simulink model "model_decouple_V0"  (R2020b)
settings: Solver=VariableStepAuto  StartTime=0.0  StopTime=10.0  RelTol=1e-3
values from neighbouring files (symbols this model uses):
  Px_e = xSeq    (= 0)    [Valeur_Equilibre.m]
  Py_e = ySeq    (= 0)    [Valeur_Equilibre.m]
  Vx_e = 0    [Valeur_Equilibre.m]
  Vy_e = 0    [Valeur_Equilibre.m]
  zD_e = Pzeq - XD*Ayeq + YD*Axeq    [Valeur_Equilibre.m]
  zE_e = Pzeq - XE*Ayeq + YE*Axeq    [Valeur_Equilibre.m]
  zF_e = Pzeq - XF*Ayeq + YF*Axeq    [Valeur_Equilibre.m]
undefined symbols (not defined in the file or in its folder): A_Ax, A_Ay, A_Az, A_Px, A_Py, B_Ax, B_Ay, B_Az, B_Px, B_Py, C_Ax, C_Ay, C_Az, C_Px, C_Py, D_Ax, D_Ay, D_Az, D_Px, D_Py, XA, XB, XC, XD, XE, XF, YB, YC, YD, YE, YF
settings Model: Creator=Alexi  LastModifiedBy=Alexi

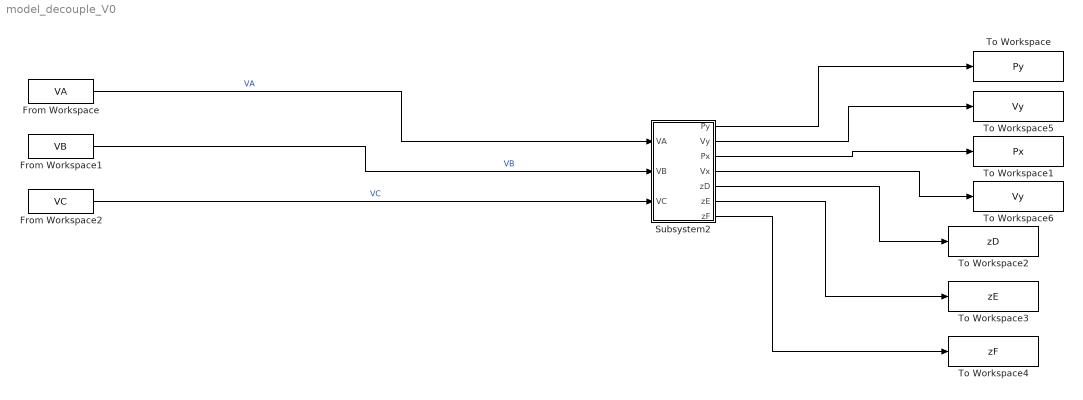
== system model_decouple_V0 ==
  From Workspace : FromWorkspace  VariableName=VA
  From Workspace1 : FromWorkspace  VariableName=VB
  From Workspace2 : FromWorkspace  VariableName=VC
  Subsystem2 : Subsystem
  To Workspace : ToWorkspace  VariableName=Py  SaveFormat=Timeseries  SampleTime=-1
  To Workspace1 : ToWorkspace  VariableName=Px  SaveFormat=Timeseries  SampleTime=-1
  To Workspace2 : ToWorkspace  VariableName=zD  SaveFormat=Timeseries  SampleTime=-1
  To Workspace3 : ToWorkspace  VariableName=zE  SaveFormat=Timeseries  SampleTime=-1
  To Workspace4 : ToWorkspace  VariableName=zF  SaveFormat=Timeseries  SampleTime=-1
  To Workspace5 : ToWorkspace  VariableName=Vy  SaveFormat=Timeseries  SampleTime=-1
  To Workspace6 : ToWorkspace  VariableName=Vy  SaveFormat=Timeseries  SampleTime=-1
  wires:
  From Workspace/1 -> Subsystem2/1(VA)  "VA"
  From Workspace1/1 -> Subsystem2/2(VB)  "VB"
  From Workspace2/1 -> Subsystem2/3(VC)  "VC"
  Subsystem2/1(Py) -> To Workspace/1
  Subsystem2/3(Px) -> To Workspace1/1
  Subsystem2/5(zD) -> To Workspace2/1
  Subsystem2/6(zE) -> To Workspace3/1
  Subsystem2/7(zF) -> To Workspace4/1
  Subsystem2/2(Vy) -> To Workspace5/1
  Subsystem2/4(Vx) -> To Workspace6/1

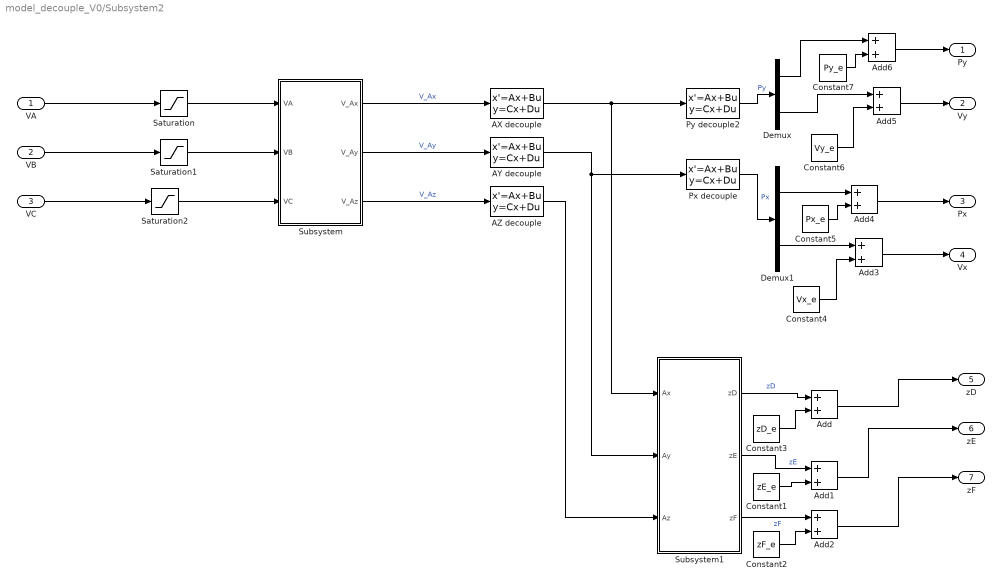
== system model_decouple_V0/Subsystem2 ==
  VA : Inport
  VB : Inport  Port=2
  VC : Inport  Port=3
  AX decouple : StateSpace  A=A_Ax  B=B_Ax  C=C_Ax  D=D_Ax  InitialCondition=0
  AY decouple : StateSpace  A=A_Ay  B=B_Ay  C=C_Ay  D=D_Ay  InitialCondition=0
  AZ decouple : StateSpace  A=A_Az  B=B_Az  C=C_Az  D=D_Az  InitialCondition=0
  Add{,1..6} (7 alike) : Sum
  Constant1 : Constant  Value=zE_e
  Constant2 : Constant  Value=zF_e
  Constant3 : Constant  Value=zD_e
  Constant4 : Constant  Value=Vx_e
  Constant5 : Constant  Value=Px_e
  Constant6 : Constant  Value=Vy_e
  Constant7 : Constant  Value=Py_e
  Demux : Demux  Outputs=2
  Demux1 : Demux  Outputs=2
  Px decouple : StateSpace  A=A_Px  B=B_Px  C=C_Px  D=D_Px  InitialCondition=0
  Py decouple2 : StateSpace  A=A_Py  B=B_Py  C=C_Py  D=D_Py  InitialCondition=0
  Saturation : Saturate  UpperLimit=22  LowerLimit=-22
  Saturation1 : Saturate  UpperLimit=22  LowerLimit=-22
  Saturation2 : Saturate  UpperLimit=22  LowerLimit=-22
  Subsystem : Subsystem
  Subsystem1 : Subsystem
  Py : Outport
  Vy : Outport  Port=2
  Px : Outport  Port=3
  Vx : Outport  Port=4
  zD : Outport  Port=5
  zE : Outport  Port=6
  zF : Outport  Port=7
  wires:
  Subsystem/2(V_Ay) -> AY decouple/1  "V_Ay"
  AX decouple/1 -> Subsystem1/1(Ax), Py decouple2/1
  Subsystem/3(V_Az) -> AZ decouple/1  "V_Az"
  Subsystem/1(V_Ax) -> AX decouple/1  "V_Ax"
  AZ decouple/1 -> Subsystem1/3(Az)
  AY decouple/1 -> Subsystem1/2(Ay), Px decouple/1
  VA/1 -> Saturation/1
  VB/1 -> Saturation1/1
  VC/1 -> Saturation2/1
  Py decouple2/1 -> Demux/1  "Py"
  Px decouple/1 -> Demux1/1  "Px"
  Subsystem1/1(zD) -> Add/1  "zD"
  Constant3/1 -> Add/2
  Constant1/1 -> Add1/2
  Subsystem1/2(zE) -> Add1/1  "zE"
  Subsystem1/3(zF) -> Add2/1  "zF"
  Constant2/1 -> Add2/2
  Add2/1 -> zF/1
  Add1/1 -> zE/1
  Add/1 -> zD/1
  Constant4/1 -> Add3/2
  Demux1/2 -> Add3/1
  Demux1/1 -> Add4/1
  Constant5/1 -> Add4/2
  Constant7/1 -> Add6/2
  Constant6/1 -> Add5/2
  Demux/1 -> Add6/1
  Demux/2 -> Add5/1
  Add6/1 -> Py/1
  Add5/1 -> Vy/1
  Add3/1 -> Vx/1
  Add4/1 -> Px/1
  Saturation/1 -> Subsystem/1(VA)
  Saturation1/1 -> Subsystem/2(VB)
  Saturation2/1 -> Subsystem/3(VC)

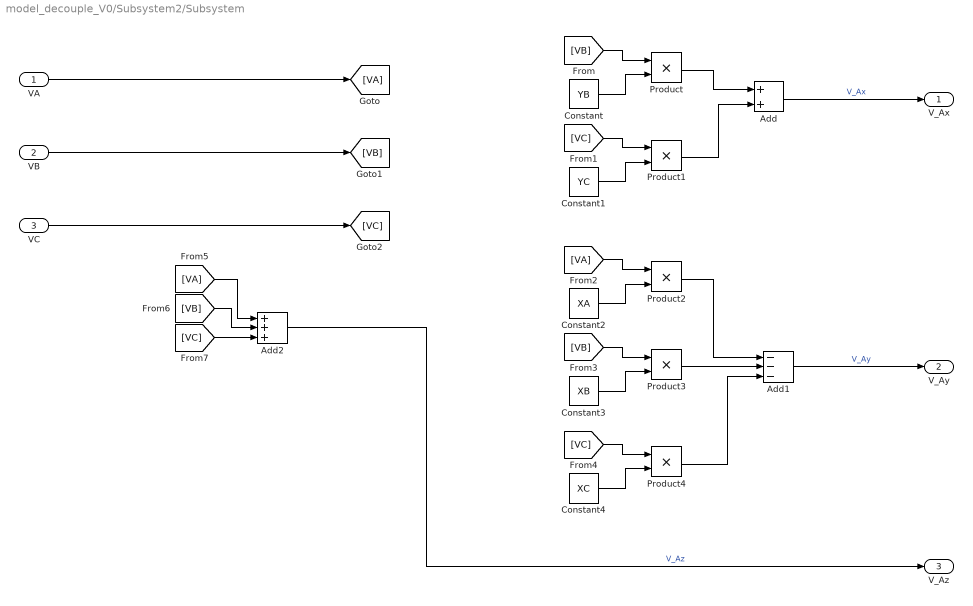
== system model_decouple_V0/Subsystem2/Subsystem ==
  VA : Inport
  VB : Inport  Port=2
  VC : Inport  Port=3
  Add : Sum
  Add1 : Sum  Inputs=---
  Add2 : Sum  Inputs=+++
  Constant : Constant  Value=YB
  Constant1 : Constant  Value=YC
  Constant2 : Constant  Value=XA
  Constant3 : Constant  Value=XB
  Constant4 : Constant  Value=XC
  Product{,1..4} (5 alike) : Product
  V_Ax : Outport
  V_Ay : Outport  Port=2
  V_Az : Outport  Port=3
  wires:
  Add2/1 -> V_Az/1  "V_Az"
  Constant4/1 -> Product4/2
  [VA] -> Add2/1
  [VC] -> Product1/1
  Product4/1 -> Add1/3
  Constant1/1 -> Product1/2
  VC/1 -> [VC]
  VA/1 -> [VA]
  Product2/1 -> Add1/1
  [VB] -> Product3/1
  [VC] -> Product4/1
  [VC] -> Add2/3
  [VB] -> Add2/2
  Constant2/1 -> Product2/2
  Constant3/1 -> Product3/2
  [VA] -> Product2/1
  Product3/1 -> Add1/2
  Product1/1 -> Add/2
  [VB] -> Product/1
  Product/1 -> Add/1
  Constant/1 -> Product/2
  VB/1 -> [VB]
  Add/1 -> V_Ax/1  "V_Ax"
  Add1/1 -> V_Ay/1  "V_Ay"

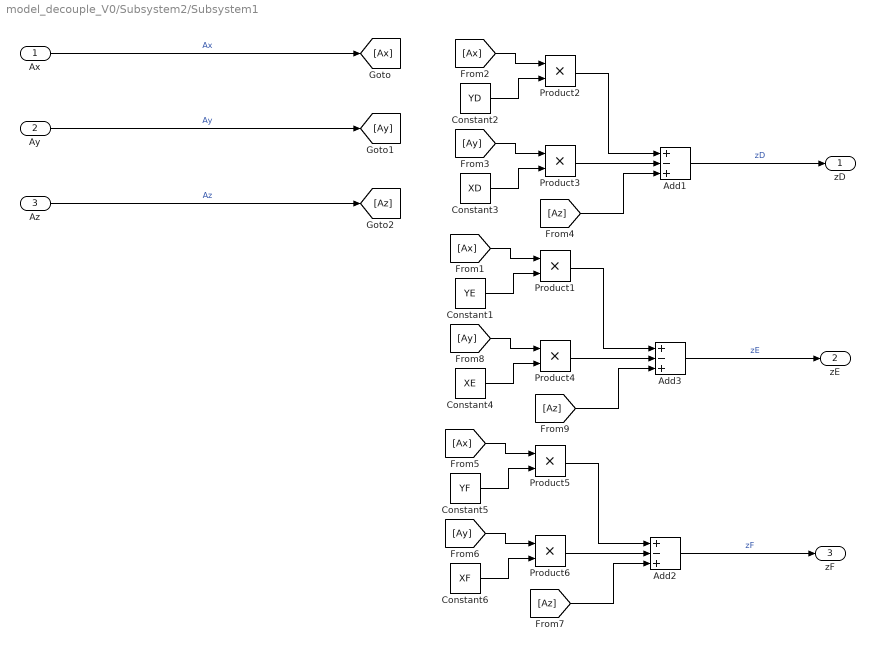
== system model_decouple_V0/Subsystem2/Subsystem1 ==
  Ax : Inport
  Ay : Inport  Port=2
  Az : Inport  Port=3
  Add1 : Sum  Inputs=+-+
  Add2 : Sum  Inputs=+-+
  Add3 : Sum  Inputs=+-+
  Constant1 : Constant  Value=YE
  Constant2 : Constant  Value=YD
  Constant3 : Constant  Value=XD
  Constant4 : Constant  Value=XE
  Constant5 : Constant  Value=YF
  Constant6 : Constant  Value=XF
  Product{1..6} (6 alike) : Product
  zD : Outport
  zE : Outport  Port=2
  zF : Outport  Port=3
  wires:
  [Az] -> Add1/3
  Az/1 -> [Az]  "Az"
  Ax/1 -> [Ax]  "Ax"
  Product2/1 -> Add1/1
  [Ay] -> Product3/1
  Constant2/1 -> Product2/2
  Constant3/1 -> Product3/2
  [Ax] -> Product2/1
  Product3/1 -> Add1/2
  Ay/1 -> [Ay]  "Ay"
  Add1/1 -> zD/1  "zD"
  Product4/1 -> Add3/2
  Constant4/1 -> Product4/2
  [Ax] -> Product1/1
  [Az] -> Add3/3
  [Ay] -> Product4/1
  Add3/1 -> zE/1  "zE"
  Constant1/1 -> Product1/2
  Product1/1 -> Add3/1
  Constant6/1 -> Product6/2
  [Az] -> Add2/3
  [Ay] -> Product6/1
  Product6/1 -> Add2/2
  Product5/1 -> Add2/1
  Constant5/1 -> Product5/2
  Add2/1 -> zF/1  "zF"
  [Ax] -> Product5/1
